simulink model "Observer"  (R2017b)
settings: Solver=VariableStepAuto  StartTime=0.0  StopTime=1  RelTol=1e-3
values from neighbouring files (symbols this model uses):
  A = [0          1                        0                0 ... (first row only)    [InvertedPendulum.m]
  B = [0; 4/(4*M+m); 0; 3/(4*M*l+m*l)]    [InvertedPendulum.m]
  C = [1 0 0 0; 0 0 1 0]    [InvertedPendulum.m]
settings Model: Creator=Daniel Ramos  LastModifiedBy=Daniel Ramos

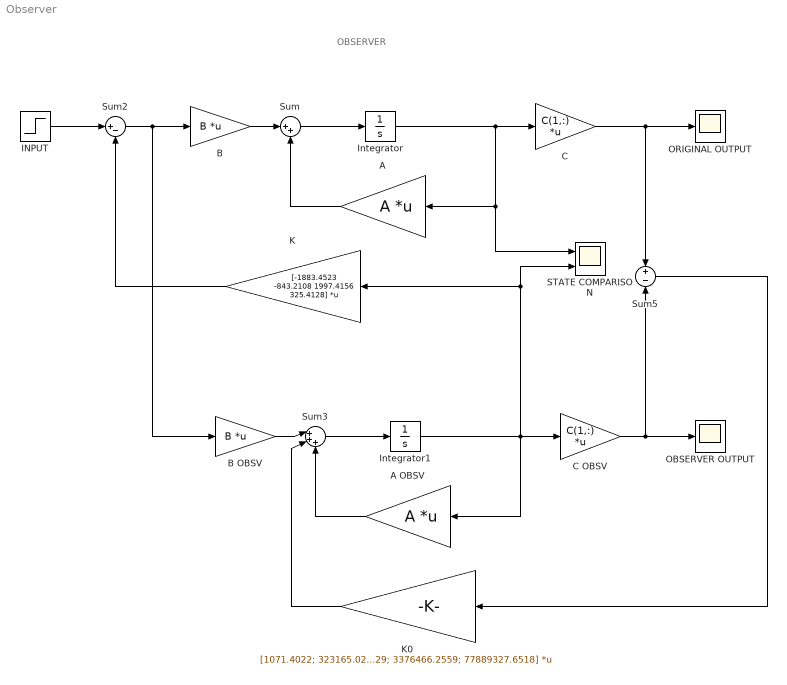
== system Observer ==
  note: OBSERVER
  A : Gain  Gain=A  Multiplication=Matrix(K*u)
  A OBSV : Gain  Gain=A  Multiplication=Matrix(K*u)
  B : Gain  Gain=B  Multiplication=Matrix(K*u)
  B OBSV : Gain  Gain=B  Multiplication=Matrix(K*u)
  C : Gain  Gain=C(1,:)  Multiplication=Matrix(K*u)
  C OBSV : Gain  Gain=C(1,:)  Multiplication=Matrix(K*u)
  INPUT : Step  Time=0  SampleTime=0
  Integrator : Integrator
  Integrator1 : Integrator  InitialCondition=[-1 -1 -1 -1]
  K : Gain  Gain=[-1883.4523 -843.2108 1997.4156 325.4128]  Multiplication=Matrix(K*u)
  K0 : Gain  Gain=[1071.4022; 323165.0229; 3376466.2559; 77889327.6518]  Multiplication=Matrix(K*u)
  OBSERVER OUTPUT : Scope
  ORIGINAL OUTPUT : Scope
  STATE COMPARISON : Scope  NumInputPorts=2
  Sum : Sum  Inputs=|++
  Sum2 : Sum  Inputs=|+-
  Sum3 : Sum  Inputs=|+++
  Sum5 : Sum  Inputs=+|-
  wires:
  A OBSV/1 -> Sum3/3
  K0/1 -> Sum3/2
  B OBSV/1 -> Sum3/1
  Sum5/1 -> K0/1
  Sum3/1 -> Integrator1/1
  Sum2/1 -> B OBSV/1, B/1
  Sum/1 -> Integrator/1
  Integrator1/1 -> STATE COMPARISON/2, K/1, A OBSV/1, C OBSV/1
  C/1 -> ORIGINAL OUTPUT/1, Sum5/1
  B/1 -> Sum/1
  C OBSV/1 -> OBSERVER OUTPUT/1, Sum5/2
  K/1 -> Sum2/2
  Integrator/1 -> STATE COMPARISON/1, A/1, C/1
  A/1 -> Sum/2
  INPUT/1 -> Sum2/1
